simulink model "Marine_LocoMotive_UAV_est_git"  (R2018a)
settings: Solver=ode4  StartTime=0.0  StopTime=40  FixedStep=T  MaxStep=2*T  MinStep=T  RelTol=1e-4
values from neighbouring files (symbols this model uses):
  a_11 = 0.05*m_b    (= 0.625)    [Marine_LocoMotive_UAV_est_git_parameters.m]    (also in Marine_LocoMotive_UAV_medium_est_git_parameters.m = 1.6875; heave_dynamics_chart.m)
  a_33 = m_b    (= 12.5)    [Marine_LocoMotive_UAV_est_git_parameters.m]    (also in Marine_LocoMotive_UAV_medium_est_git_parameters.m = 33.75; heave_dynamics_chart.m)
  A_w = 1*3.3/2    (= 1.65)    [Marine_LocoMotive_UAV_est_git_parameters.m]    (also in Marine_LocoMotive_UAV_medium_est_git_parameters.m = 0.6)
  A_w2 = 1*1.2/2    (= 0.6)    [Marine_LocoMotive_UAV_est_git_parameters.m]    (also in Marine_LocoMotive_UAV_medium_est_git_parameters.m = 0.305)
  Ac = 0.0331    [Marine_LocoMotive_UAV_est_git_parameters.m]    (also in Marine_LocoMotive_UAV_medium_est_git_parameters.m = 0.422)
  alpha_bar = pi/4    (= 0.785398163397)    [Marine_LocoMotive_UAV_est_git_parameters.m]    (also in Marine_LocoMotive_UAV_medium_est_git_parameters.m; heave_dynamics_chart.m = pi/4*sign(V_bar(j)))
  Am = sysd.denominator{1}    [Marine_LocoMotive_UAV_est_git_parameters.m]    (also in Marine_LocoMotive_UAV_medium_est_git_parameters.m)
  Am1_LPF = sysd.denominator{1}    [Marine_LocoMotive_UAV_est_git_parameters.m]    (also in Marine_LocoMotive_UAV_medium_est_git_parameters.m)
  Am2_LPF = sysd.denominator{1}    [Marine_LocoMotive_UAV_est_git_parameters.m]    (also in Marine_LocoMotive_UAV_medium_est_git_parameters.m)
  Am_asw_LPF = sysd.denominator{1}    [Marine_LocoMotive_UAV_est_git_parameters.m]    (also in Marine_LocoMotive_UAV_medium_est_git_parameters.m)
  Am_coup_LPF = sysd.denominator{1}    [Marine_LocoMotive_UAV_est_git_parameters.m]    (also in Marine_LocoMotive_UAV_medium_est_git_parameters.m)
  Am_fast_coup_LPF = sysd.denominator{1}    [Marine_LocoMotive_UAV_est_git_parameters.m]    (also in Marine_LocoMotive_UAV_medium_est_git_parameters.m)
  Am_rdeL_LPF = sysd.denominator{1}    [Marine_LocoMotive_UAV_est_git_parameters.m]    (also in Marine_LocoMotive_UAV_medium_est_git_parameters.m)
  Am_reL_LPF = sysd.denominator{1}    [Marine_LocoMotive_UAV_est_git_parameters.m]    (also in Marine_LocoMotive_UAV_medium_est_git_parameters.m)
  Am_rref20_LPF = sysd.denominator{1}    [Marine_LocoMotive_UAV_est_git_parameters.m]    (also in Marine_LocoMotive_UAV_medium_est_git_parameters.m)
  Am_rref_LPF = sysd.denominator{1}    [Marine_LocoMotive_UAV_est_git_parameters.m]    (also in Marine_LocoMotive_UAV_medium_est_git_parameters.m)
  AmAlpha_LPF = sysd.denominator{1}    [Marine_LocoMotive_UAV_est_git_parameters.m]    (also in Marine_LocoMotive_UAV_medium_est_git_parameters.m)
  Amp_sf = 3    [Marine_LocoMotive_UAV_est_git_parameters.m]    (also in Marine_LocoMotive_UAV_medium_est_git_parameters.m)
  Amp_sf_rp = 0.05*m_u*g    (= 0.8829)    [Marine_LocoMotive_UAV_est_git_parameters.m]    (also in Marine_LocoMotive_UAV_medium_est_git_parameters.m = 9.56475)
  AmV_LPF = sysd.denominator{1}    [Marine_LocoMotive_UAV_est_git_parameters.m]    (also in Marine_LocoMotive_UAV_medium_est_git_parameters.m)
  AmZ_LPF = sysd.denominator{1}    [Marine_LocoMotive_UAV_est_git_parameters.m]    (also in Marine_LocoMotive_UAV_medium_est_git_parameters.m)
  b_11 = 0    [Marine_LocoMotive_UAV_est_git_parameters.m]    (also in Marine_LocoMotive_UAV_medium_est_git_parameters.m; heave_dynamics_chart.m)
  b_33 = 2*m_b*omega_h    (= 19.6349540849)    [Marine_LocoMotive_UAV_est_git_parameters.m]    (also in Marine_LocoMotive_UAV_medium_est_git_parameters.m = 84.8230016469; buoyancy_calc.m = 4.18879020479; heave_dynamics_chart.m = 2*m_b*omega_h)
  Bm = sysd.numerator{1}    [Marine_LocoMotive_UAV_est_git_parameters.m]    (also in Marine_LocoMotive_UAV_medium_est_git_parameters.m)
  Bm1_LPF = sysd.numerator{1}    [Marine_LocoMotive_UAV_est_git_parameters.m]    (also in Marine_LocoMotive_UAV_medium_est_git_parameters.m)
  Bm2_LPF = sysd.numerator{1}    [Marine_LocoMotive_UAV_est_git_parameters.m]    (also in Marine_LocoMotive_UAV_medium_est_git_parameters.m)
  Bm_asw_LPF = sysd.numerator{1}    [Marine_LocoMotive_UAV_est_git_parameters.m]    (also in Marine_LocoMotive_UAV_medium_est_git_parameters.m)
  Bm_coup_LPF = sysd.numerator{1}    [Marine_LocoMotive_UAV_est_git_parameters.m]    (also in Marine_LocoMotive_UAV_medium_est_git_parameters.m)
  Bm_fast_coup_LPF = sysd.numerator{1}    [Marine_LocoMotive_UAV_est_git_parameters.m]    (also in Marine_LocoMotive_UAV_medium_est_git_parameters.m)
  Bm_rdeL_LPF = sysd.numerator{1}    [Marine_LocoMotive_UAV_est_git_parameters.m]    (also in Marine_LocoMotive_UAV_medium_est_git_parameters.m)
  Bm_reL_LPF = sysd.numerator{1}    [Marine_LocoMotive_UAV_est_git_parameters.m]    (also in Marine_LocoMotive_UAV_medium_est_git_parameters.m)
  Bm_rref20_LPF = sysd.numerator{1}    [Marine_LocoMotive_UAV_est_git_parameters.m]    (also in Marine_LocoMotive_UAV_medium_est_git_parameters.m)
  Bm_rref_LPF = sysd.numerator{1}    [Marine_LocoMotive_UAV_est_git_parameters.m]    (also in Marine_LocoMotive_UAV_medium_est_git_parameters.m)
  BmAlpha_LPF = sysd.numerator{1}    [Marine_LocoMotive_UAV_est_git_parameters.m]    (also in Marine_LocoMotive_UAV_medium_est_git_parameters.m)
  BmV_LPF = sysd.numerator{1}    [Marine_LocoMotive_UAV_est_git_parameters.m]    (also in Marine_LocoMotive_UAV_medium_est_git_parameters.m)
  BmZ_LPF = sysd.numerator{1}    [Marine_LocoMotive_UAV_est_git_parameters.m]    (also in Marine_LocoMotive_UAV_medium_est_git_parameters.m)
  C_S = [5;9]*10^-3    [Marine_LocoMotive_UAV_est_git_parameters.m]    (also in Marine_LocoMotive_UAV_medium_est_git_parameters.m; heave_dynamics_chart.m = 0.075/(log10(Re)-2)^2)
  Cd_u = 0.2    [Marine_LocoMotive_UAV_est_git_parameters.m]    (also in Marine_LocoMotive_UAV_medium_est_git_parameters.m)
  D_x = b_11 + D_s(1)    [Marine_LocoMotive_UAV_est_git_parameters.m]    (also in Marine_LocoMotive_UAV_medium_est_git_parameters.m; heave_dynamics_chart.m = b_11 + D_s(i,j))
  D_z = b_33 + D_s(2)    [Marine_LocoMotive_UAV_est_git_parameters.m]    (also in Marine_LocoMotive_UAV_medium_est_git_parameters.m; heave_dynamics_chart.m)
  dc_M_p = 6.7    [Marine_LocoMotive_UAV_est_git_parameters.m]    (also in Marine_LocoMotive_UAV_medium_est_git_parameters.m)
  Delta_h = (A_im/A_b-0.5)*h_b    (= -0.0625)    [Marine_LocoMotive_UAV_est_git_parameters.m]    (also in Marine_LocoMotive_UAV_medium_est_git_parameters.m = -0.075; heave_dynamics_chart.m)
  eps_V = 0.1    [Marine_LocoMotive_UAV_est_git_parameters.m]    (also in Marine_LocoMotive_UAV_medium_est_git_parameters.m)
  epsilon_1 = 5    [Marine_LocoMotive_UAV_est_git_parameters.m]    (also in Marine_LocoMotive_UAV_medium_est_git_parameters.m)
  epsilon_e_u1 = 0.05    [Marine_LocoMotive_UAV_est_git_parameters.m]    (also in Marine_LocoMotive_UAV_medium_est_git_parameters.m)
  epsilon_w = 0    [Marine_LocoMotive_UAV_est_git_parameters.m]    (also in Marine_LocoMotive_UAV_medium_est_git_parameters.m)
  epsilon_w2 = pi    (= 3.14159265359)    [Marine_LocoMotive_UAV_est_git_parameters.m]    (also in Marine_LocoMotive_UAV_medium_est_git_parameters.m)
  g = 9.81    [Marine_LocoMotive_UAV_est_git_parameters.m]    (also in Marine_LocoMotive_UAV_medium_est_git_parameters.m; heave_dynamics_chart.m)
  gamma_d_p = (2*0.3/0.03*2*0.2*12/4)/10    (= 2.4)    [Marine_LocoMotive_UAV_est_git_parameters.m]    (also in Marine_LocoMotive_UAV_medium_est_git_parameters.m)
  H = 10    [Marine_LocoMotive_UAV_est_git_parameters.m]    (also in Marine_LocoMotive_UAV_medium_est_git_parameters.m)
  h_b = 0.25    [Marine_LocoMotive_UAV_est_git_parameters.m]    (also in Marine_LocoMotive_UAV_medium_est_git_parameters.m = 0.3; buoyancy_calc.m = 0.15; heave_dynamics_chart.m)
  J_b = m_b*h_b*l_b/12    (= 0.208333333333)    [Marine_LocoMotive_UAV_est_git_parameters.m]    (also in Marine_LocoMotive_UAV_medium_est_git_parameters.m = 1.265625; heave_dynamics_chart.m)
  J_u = 0.03    [Marine_LocoMotive_UAV_est_git_parameters.m]    (also in Marine_LocoMotive_UAV_medium_est_git_parameters.m = 1.51708333333)
  K = 40    [Marine_LocoMotive_UAV_est_git_parameters.m]    (also in Marine_LocoMotive_UAV_medium_est_git_parameters.m = 83.3333333333)
  k3 = 24    [Marine_LocoMotive_UAV_est_git_parameters.m]    (also in Marine_LocoMotive_UAV_medium_est_git_parameters.m)
  k4 = 0.8    [Marine_LocoMotive_UAV_est_git_parameters.m]    (also in Marine_LocoMotive_UAV_medium_est_git_parameters.m)
  k_w = omega_w^2/g    (= 0.0628797426165)    [Marine_LocoMotive_UAV_est_git_parameters.m]    (also in Marine_LocoMotive_UAV_medium_est_git_parameters.m = 0.160972141098; heave_dynamics_chart.m = omega_w^2/g)
  k_w2 = omega_w2^2/g    (= 0.160972141098)    [Marine_LocoMotive_UAV_est_git_parameters.m]    (also in Marine_LocoMotive_UAV_medium_est_git_parameters.m = 0.251518970466)
  kd_a = 5.6    [Marine_LocoMotive_UAV_est_git_parameters.m]    (also in Marine_LocoMotive_UAV_medium_est_git_parameters.m)
  kd_r = 19.5    [Marine_LocoMotive_UAV_est_git_parameters.m]    (also in Marine_LocoMotive_UAV_medium_est_git_parameters.m)
  kd_t = 10    [Marine_LocoMotive_UAV_est_git_parameters.m]    (also in Marine_LocoMotive_UAV_medium_est_git_parameters.m = 25)
  kd_x = 5    [Marine_LocoMotive_UAV_est_git_parameters.m]    (also in Marine_LocoMotive_UAV_medium_est_git_parameters.m)
  kd_z = 2    [Marine_LocoMotive_UAV_est_git_parameters.m]    (also in Marine_LocoMotive_UAV_medium_est_git_parameters.m)
  ki_a = 1.6    [Marine_LocoMotive_UAV_est_git_parameters.m]    (also in Marine_LocoMotive_UAV_medium_est_git_parameters.m)
  ki_r = 9    [Marine_LocoMotive_UAV_est_git_parameters.m]    (also in Marine_LocoMotive_UAV_medium_est_git_parameters.m)
  ki_T = 12    [Marine_LocoMotive_UAV_est_git_parameters.m]    (also in Marine_LocoMotive_UAV_medium_est_git_parameters.m)
  ki_x = 1.2    [Marine_LocoMotive_UAV_est_git_parameters.m]    (also in Marine_LocoMotive_UAV_medium_est_git_parameters.m)
  ki_z = 1    [Marine_LocoMotive_UAV_est_git_parameters.m]    (also in Marine_LocoMotive_UAV_medium_est_git_parameters.m)
  kp_a = 9.6    [Marine_LocoMotive_UAV_est_git_parameters.m]    (also in Marine_LocoMotive_UAV_medium_est_git_parameters.m)
  kp_r = 45    [Marine_LocoMotive_UAV_est_git_parameters.m]    (also in Marine_LocoMotive_UAV_medium_est_git_parameters.m)
  kp_t = 20    [Marine_LocoMotive_UAV_est_git_parameters.m]    (also in Marine_LocoMotive_UAV_medium_est_git_parameters.m = 50)
  kp_T = 25    [Marine_LocoMotive_UAV_est_git_parameters.m]    (also in Marine_LocoMotive_UAV_medium_est_git_parameters.m)
  kp_x = 7    [Marine_LocoMotive_UAV_est_git_parameters.m]    (also in Marine_LocoMotive_UAV_medium_est_git_parameters.m)
  kp_z = 3    [Marine_LocoMotive_UAV_est_git_parameters.m]    (also in Marine_LocoMotive_UAV_medium_est_git_parameters.m)
  L = 0.2    [Marine_LocoMotive_UAV_est_git_parameters.m]    (also in Marine_LocoMotive_UAV_medium_est_git_parameters.m = 0.8)
  l_b = 0.8    [Marine_LocoMotive_UAV_est_git_parameters.m]    (also in Marine_LocoMotive_UAV_medium_est_git_parameters.m = 1.5; buoyancy_calc.m = 0.5; heave_dynamics_chart.m)
  Lc_0 = 7    [Marine_LocoMotive_UAV_est_git_parameters.m]    (also in Marine_LocoMotive_UAV_medium_est_git_parameters.m = 20)
  LIMIT_CMD_PITCH = 45*pi/180    (= 0.785398163397)    [Marine_LocoMotive_UAV_est_git_parameters.m]    (also in Marine_LocoMotive_UAV_medium_est_git_parameters.m)
  LIMIT_uCMD_HEIGHT = 0.9*n_motors*K    (= 144)    [Marine_LocoMotive_UAV_est_git_parameters.m]    (also in Marine_LocoMotive_UAV_medium_est_git_parameters.m = 450)
  m_b = rho_w*Vol_b/4    (= 12.5)    [Marine_LocoMotive_UAV_est_git_parameters.m]    (also in Marine_LocoMotive_UAV_medium_est_git_parameters.m = 33.75; buoyancy_calc.m = 5; heave_dynamics_chart.m)
  m_u = 1.8    [Marine_LocoMotive_UAV_est_git_parameters.m]    (also in Marine_LocoMotive_UAV_medium_est_git_parameters.m = 19.5)
  min_sf = 5    [Marine_LocoMotive_UAV_est_git_parameters.m]    (also in Marine_LocoMotive_UAV_medium_est_git_parameters.m)
  min_sf_rp = 0.35*m_u*g    (= 6.1803)    [Marine_LocoMotive_UAV_est_git_parameters.m]    (also in Marine_LocoMotive_UAV_medium_est_git_parameters.m = 66.95325)
  n_motors = 4    [Marine_LocoMotive_UAV_est_git_parameters.m]    (also in Marine_LocoMotive_UAV_medium_est_git_parameters.m = 6)
  nu_w = 1.787*10^-6    (= 1.787e-06)    [Marine_LocoMotive_UAV_est_git_parameters.m]    (also in Marine_LocoMotive_UAV_medium_est_git_parameters.m; buoyancy_calc.m; heave_dynamics_chart.m)
  omega_w = 2*pi/T_w    (= 0.785398163397)    [Marine_LocoMotive_UAV_est_git_parameters.m]    (also in Marine_LocoMotive_UAV_medium_est_git_parameters.m = 1.25663706144; heave_dynamics_chart.m = 2*pi/T_i)
  omega_w2 = 2*pi/T_w2    (= 1.25663706144)    [Marine_LocoMotive_UAV_est_git_parameters.m]    (also in Marine_LocoMotive_UAV_medium_est_git_parameters.m = 1.57079632679)
  r_0 = sqrt( (X0_b(1) - X0_u(1))^2 +(X0_b(2) - X0_u(2))^2 )    [Marine_LocoMotive_UAV_est_git_parameters.m]    (also in Marine_LocoMotive_UAV_medium_est_git_parameters.m)
  R_b = 0.1    [buoyancy_calc.m]
  r_bar = Lc_0-0.3    (= 6.7)    [Marine_LocoMotive_UAV_est_git_parameters.m]    (also in Marine_LocoMotive_UAV_medium_est_git_parameters.m = 19.7)
  r_min = (zu_bar-H)-0.2    [Marine_LocoMotive_UAV_est_git_parameters.m]    (also in Marine_LocoMotive_UAV_medium_est_git_parameters.m)
  rho_a = 1.225    [Marine_LocoMotive_UAV_est_git_parameters.m]    (also in Marine_LocoMotive_UAV_medium_est_git_parameters.m)
  rho_w = 1000    [Marine_LocoMotive_UAV_est_git_parameters.m]    (also in Marine_LocoMotive_UAV_medium_est_git_parameters.m; buoyancy_calc.m; heave_dynamics_chart.m)
  T = 1/500    (= 0.002)    [Marine_LocoMotive_UAV_est_git_parameters.m]    (also in Marine_LocoMotive_UAV_medium_est_git_parameters.m)
  T_init = 10    [Marine_LocoMotive_UAV_est_git_parameters.m]    (also in Marine_LocoMotive_UAV_medium_est_git_parameters.m)
  Theta0 = 0    [Marine_LocoMotive_UAV_est_git_parameters.m]    (also in Marine_LocoMotive_UAV_medium_est_git_parameters.m)
  torque_corr = 2*cosd(60)+1    [Marine_LocoMotive_UAV_est_git_parameters.m]    (also in Marine_LocoMotive_UAV_medium_est_git_parameters.m)
  u_s = w_dir*A_w^2*omega_w*k_w*exp(2*k_w*(-Delta_h/2))    [Marine_LocoMotive_UAV_est_git_parameters.m]    (also in Marine_LocoMotive_UAV_medium_est_git_parameters.m)
  u_s2 = w_dir2*A_w2^2*omega_w2*k_w2*exp(2*k_w2*(-Delta_h/2))    [Marine_LocoMotive_UAV_est_git_parameters.m]    (also in Marine_LocoMotive_UAV_medium_est_git_parameters.m)
  u_t = -1*0.5*1    (= -0.5)    [Marine_LocoMotive_UAV_est_git_parameters.m]    (also in Marine_LocoMotive_UAV_medium_est_git_parameters.m)
  u_w = 0*0.2    (= 0)    [Marine_LocoMotive_UAV_est_git_parameters.m]    (also in Marine_LocoMotive_UAV_medium_est_git_parameters.m)
  V0_b = [u_t+u_w+u_s+v_x_w, v_z_w].*[1 1]    [Marine_LocoMotive_UAV_est_git_parameters.m]    (also in Marine_LocoMotive_UAV_medium_est_git_parameters.m = [u_t+u_w+u_s+v_x_w, v_z_w])
  V0_u = V0_b    [Marine_LocoMotive_UAV_est_git_parameters.m]    (also in Marine_LocoMotive_UAV_medium_est_git_parameters.m = [0 0])
  V_bar = 4    [Marine_LocoMotive_UAV_est_git_parameters.m]    (also in Marine_LocoMotive_UAV_medium_est_git_parameters.m; heave_dynamics_chart.m = [-20:0.1:20]')
  Vol_b = A_b*l_b    (= 0.05)    [Marine_LocoMotive_UAV_est_git_parameters.m]    (also in Marine_LocoMotive_UAV_medium_est_git_parameters.m = 0.135; heave_dynamics_chart.m)
  w_dir = 1    [Marine_LocoMotive_UAV_est_git_parameters.m]    (also in Marine_LocoMotive_UAV_medium_est_git_parameters.m; heave_dynamics_chart.m)
  w_dir2 = 1    [Marine_LocoMotive_UAV_est_git_parameters.m]    (also in Marine_LocoMotive_UAV_medium_est_git_parameters.m)
  X0_b = [0,H-Delta_h]    [Marine_LocoMotive_UAV_est_git_parameters.m]    (also in Marine_LocoMotive_UAV_medium_est_git_parameters.m)
  X0_u = X0_b + [3/7 3/7]*Lc_0    [Marine_LocoMotive_UAV_est_git_parameters.m]    (also in Marine_LocoMotive_UAV_medium_est_git_parameters.m)
  zu_bar = X0_b(2) + Lc_0*sin(alpha_bar_0)    [Marine_LocoMotive_UAV_est_git_parameters.m]    (also in Marine_LocoMotive_UAV_medium_est_git_parameters.m)
undefined symbols (not defined in the file or in its folder): Am_HPF, Am_LPF, Am_LPF2, an1, an1_v, an2, an3, Bm_HPF, Bm_LPF, Bm_LPF2, bn1, bn1_v, bn2, bn3, DiscIntNeverNeededParam, F, Light, magnitude, MIL, OMEGA_FILTER_OUTER, Tc, Tg, Tn, Ts, Tsc, Tz, X_GPS_offset
libraries: simulink x55, simulink_extras x9, aerolibwind2 x2
(part 2 of 9)

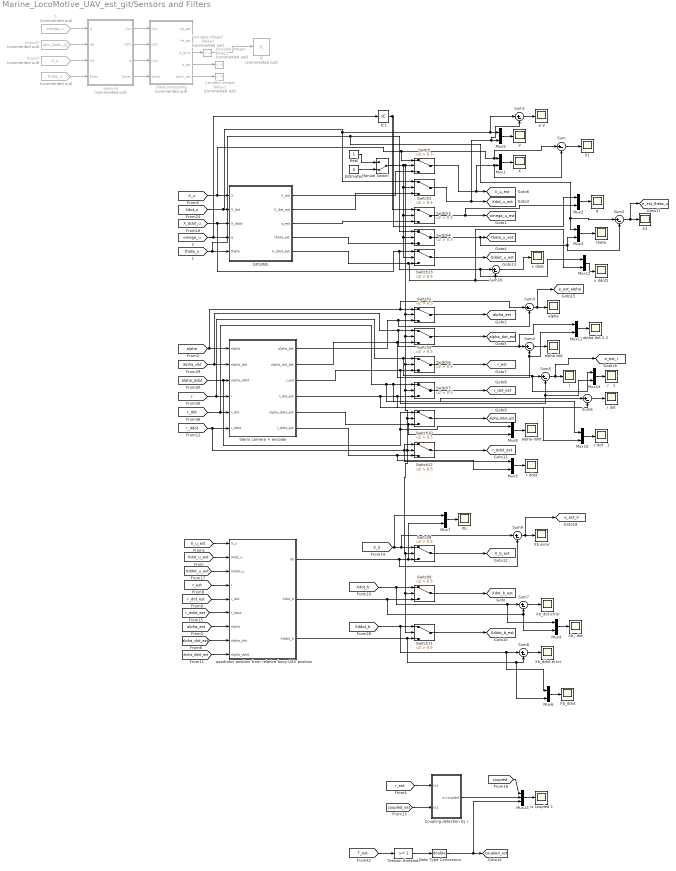
== system Marine_LocoMotive_UAV_est_git/Sensors and Filters ==
  "    " : From  Commented=on  GotoTag=theta_u  TagVisibility=global
  "   1" : From  Commented=on  GotoTag=omega_u  TagVisibility=global
  Coupling detection by r : Subsystem
  Data Type Conversion : DataTypeConversion  OutDataTypeStr=double
  Data processing : Subsystem  Commented=on
  Estimates : Constant  Value=0
  From37 : From  Commented=on  GotoTag=acc_body_u  TagVisibility=global
  From7 : From  Commented=on  GotoTag=X_u  TagVisibility=global
  GPS/INS : Subsystem
  IC : InitialCondition  Commented=on  Value=0
  IC1 : InitialCondition  Value=0
  Manual Switch : ManualSwitch  CurrentSetting=0
  Mux{1..12,14} (13 alike) : Mux  Inputs=2
  Mux13 : Mux  Inputs=3
  Real : Constant
  Sensors : Subsystem  Commented=on
  Sterio camera + encoder : Subsystem
  Sum{,1..10} (11 alike) : Sum  Inputs=|+-
  Switch{,1..13} (14 alike) : Switch  Criteria=u2 > Threshold  Threshold=0.5
  Tension threshold : simulink/Logic and Bit Operations/Compare To Constant  relop=>=  const=1  OutDataTypeStr=boolean
  V : Scope
  Variable Integer Delay1 : Delay  Commented=on  DelayLength=0
  Variable Integer Delay2 : Delay  Commented=on  DelayLength=0
  Variable Integer Delay3 : Delay  Commented=on  DelayLength=0
  X : Scope
  X1 : Scope
  X3 : Scope
  "Xb " : Scope
  Xb error : Scope
  "Xb_ dot " : Scope
  "Xb_ddot " : Scope
  "Xb_ddot error  " : Scope
  Xb_dot error : Scope
  "alpha  " : Scope
  "alpha ddot " : Scope
  "alpha dot " : Scope
  alpha dot 2 2 : Scope
  e V : Scope
  is coupled 1 : Scope
  q : Scope
  quadrotor position from relative buoy-UAV position : Subsystem
  "r   " : Scope
  r   1 : Scope
  "r ddot   " : Scope
  "r dot  " : Scope
  r dot   1 : Scope
  theta : Scope
  x ddot : Scope
  x ddot1 : Scope
  tag scope: X_b_est=global, X_u_est=global, Xddot_b_est=global, Xddot_u_est=global, Xdot_b_est=global, Xdot_u_est=global, alpha_ddot_est=global, alpha_dot_est=global, alpha_est=global, coupled_est=global, e_est_V=global, e_est_alpha=global, e_est_r=global, e_est_theta_u=global, omega_u_est=global, r_ddot_est=global, r_dot_est=global, r_est=global, theta_u_est=global
  wires:
  Data processing/4("q_est ") -> Variable Integer Delay1/1
  "    "/1 -> Sensors/4(Euler)
  Sensors/3(" q") -> Data processing/3(p,q,r)
  "   1"/1 -> Sensors/1("q ")
  From7/1 -> Sensors/3(Xe)
  Sensors/1(Acc) -> Data processing/1(Acc)
  Sensors/2(GPS) -> Data processing/2("GPS ")
  From37/1 -> Sensors/2(Ab)
  Data processing/3(q_gyro) -> Variable Integer Delay3/1
  Data processing/5(pitch_est) -> Variable Integer Delay2/1
  Sensors/4(Sonar) -> Data processing/4(Sonar)
  Estimates/1 -> Manual Switch/2
  Real/1 -> Manual Switch/1
  Switch/1 -> Sum/2, Mux1/2, [X_u_est]
  Switch1/1 -> Sum1/2, Mux5/2, [Xdot_u_est]
  Switch3/1 -> Mux2/2, [omega_u_est]
  Switch4/1 -> Mux3/2, Sum2/2, [theta_u_est]
  GPS/INS/1(X_est) -> Switch/3
  GPS/INS/2(X_dot_est) -> Switch1/3
  Variable Integer Delay3/1 -> IC/1
  [X_u] -> Sum/1, Mux1/1, Switch/1, GPS/INS/1(X)
  [omega_u] -> IC1/1, GPS/INS/4(q)
  [Xdot_u] -> Sum1/1, Mux5/1, Switch1/1, GPS/INS/2(X_dot)
  GPS/INS/4(theta_est) -> Switch4/3
  GPS/INS/3(q_est) -> Switch3/3
  IC1/1 -> Mux2/1, Switch3/1
  [theta_u] -> Sum2/1, Mux3/1, Switch4/1, GPS/INS/5(theta)
  Mux5/1 -> V/1
  Mux1/1 -> X/1
  Mux2/1 -> q/1
  Mux3/1 -> theta/1
  Sum/1 -> X1/1
  Sum1/1 -> e V/1
  Sum2/1 -> [e_est_theta_u], X3/1
  [alpha_dot] -> Mux11/1, Sum4/1, Switch5/1, Sterio camera + encoder/2(alpha_dot)
  [r] -> Mux14/1, Sum5/1, Switch6/1, Sterio camera + encoder/4(r)
  [r_dot] -> Mux10/1, Sum6/1, Switch7/1, Sterio camera + encoder/5(r_dot)
  Sterio camera + encoder/2(alpha_dot_est) -> Mux11/2, Sum4/2, Switch5/3
  Sterio camera + encoder/3(r_est) -> Sum5/2, Mux14/2, Switch6/3
  Switch2/1 -> [alpha_est]
  Switch5/1 -> [alpha_dot_est]
  Switch6/1 -> [r_est]
  Switch7/1 -> [r_dot_est]
  Sum3/1 -> [e_est_alpha], "alpha  "/1
  [alpha] -> Sum3/1, Switch2/1, Sterio camera + encoder/1(alpha)
  Sterio camera + encoder/1(alpha_est) -> Sum3/2, Switch2/3
  Sum4/1 -> "alpha dot "/1
  Sum5/1 -> [e_est_r], "r   "/1
  Sterio camera + encoder/4(r_dot_est) -> Mux10/2, Sum6/2, Switch7/3
  Sum6/1 -> "r dot  "/1
  [X_u_est] -> quadrotor position from relative buoy-UAV position/1(X_u)
  [Xdot_u_est] -> quadrotor position from relative buoy-UAV position/2(Xdot_u)
  [r_est] -> quadrotor position from relative buoy-UAV position/4(r)
  [r_dot_est] -> quadrotor position from relative buoy-UAV position/5(r_dot)
  [alpha_est] -> quadrotor position from relative buoy-UAV position/7(alpha)
  [alpha_dot_est] -> quadrotor position from relative buoy-UAV position/8(alpha_dot)
  quadrotor position from relative buoy-UAV position/2(Xdot_b) -> Mux4/2, Sum7/2, Switch9/3
  quadrotor position from relative buoy-UAV position/1(Xb) -> Sum9/2, Mux7/2, Switch8/3
  [alpha_ddot] -> Switch10/1, Mux8/1, Sterio camera + encoder/3(alpha_ddot)
  Sterio camera + encoder/5(alpha_ddot_est) -> Mux8/2, Switch10/3
  Switch10/1 -> [alpha_ddot_est]
  [Xdot_b] -> Mux4/1, Sum7/1, Switch9/1
  [alpha_ddot_est] -> quadrotor position from relative buoy-UAV position/9(alpha_ddot)
  [Xddot_u_est] -> quadrotor position from relative buoy-UAV position/3(Xddot_u)
  quadrotor position from relative buoy-UAV position/3(Xddot_b) -> Mux6/2, Sum8/2, Switch11/3
  [r_ddot] -> Mux9/1, Switch12/1, Sterio camera + encoder/6(r_ddot)
  Switch12/1 -> [r_ddot_est]
  Switch9/1 -> [Xdot_b_est]
  Switch11/1 -> [Xddot_b_est]
  Sum7/1 -> Xb_dot error/1
  Manual Switch/1 -> Switch10/2, Switch12/2, Switch8/2, Switch11/2, Switch9/2, Switch7/2, Switch6/2, Switch5/2, Switch2/2, Switch/2, Switch13/2, Switch4/2, Switch3/2, Switch1/2
  Sum8/1 -> "Xb_ddot error  "/1
  Sum9/1 -> [e_est_V], Xb error/1
  Switch8/1 -> [X_b_est]
  [X_b] -> Mux7/1, Sum9/1, Switch8/1
  Mux4/1 -> "Xb_ dot "/1
  Mux6/1 -> "Xb_ddot "/1
  [Xddot_b] -> Mux6/1, Sum8/1, Switch11/1
  [r_ddot_est] -> quadrotor position from relative buoy-UAV position/6(r_ddot)
  [X_ddot_u] -> Mux12/1, Sum10/1, Switch13/1, GPS/INS/3(X_ddot)
  Switch13/1 -> [Xddot_u_est]
  Mux7/1 -> "Xb "/1
  Mux8/1 -> "alpha ddot "/1
  Mux9/1 -> "r ddot   "/1
  Sterio camera + encoder/6(r_ddot_est) -> Mux9/2, Switch12/3
  Sum10/1 -> x ddot/1
  Mux10/1 -> r dot   1/1
  Mux11/1 -> alpha dot 2 2/1
  GPS/INS/5(X_ddot_est) -> Mux12/2, Sum10/2, Switch13/3
  Mux12/1 -> x ddot1/1
  Mux13/1 -> is coupled 1/1
  Mux14/1 -> r   1/1
  [r_est] -> Coupling detection by r/1(In1)
  [coupled_est] -> Coupling detection by r/2(In2)
  [T_est] -> Tension threshold/1
  Tension threshold/1 -> Data Type Conversion/1
  Data Type Conversion/1 -> Mux13/3, [coupled_est]
  Coupling detection by r/1(is coupled) -> Mux13/2
  [coupled] -> Mux13/1

== system Marine_LocoMotive_UAV_est_git/Subsystem ==

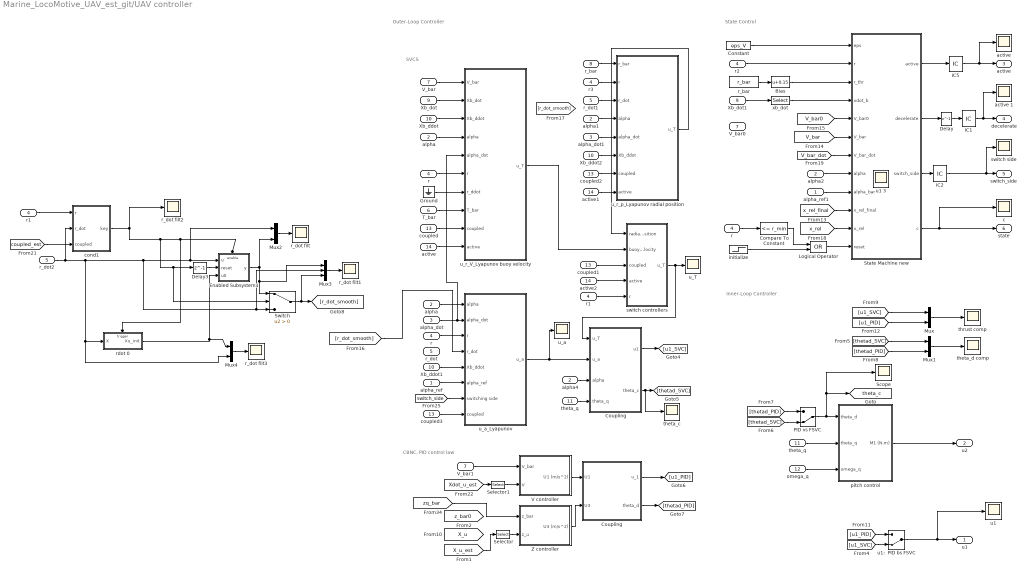
== system Marine_LocoMotive_UAV_est_git/UAV controller ==
  note: State Control
  note: Inner-Loop Controller
  note: Outer-Loop Controller
  note: CBNC, PID control law
  note: SVCS
  alpha_ref : Inport
  alpha : Inport  Port=2
  alpha_dot : Inport  Port=3
  r : Inport  Port=4
  r_dot : Inport  Port=5
  T_bar : Inport  Port=6
  V_bar : Inport  Port=7
  r_bar : Inport  Port=8
  Xb_dot : Inport  Port=9
  Xb_ddot : Inport  Port=10
  theta_q : Inport  Port=11
  omega_q : Inport  Port=12
  coupled : Inport  Port=13
  active : Inport  Port=14
  " active " : Scope
  " active 1" : Scope
  " c " : Scope
  " r" : InportShadow  Port=4
  " r1" : InportShadow  Port=4
  Bias : Bias  Bias=0.15
  Compare To Constant : simulink/Logic and Bit Operations/Compare To Constant  relop=<=  const=r_min  OutDataTypeStr=boolean
  Constant : Constant  Value=eps_V
  Coupling : Subsystem
  "Coupling " : Subsystem
  Delay : Delay  DelayLength=1  InitialCondition=0
  Delay3 : Delay  DelayLength=1  InitialCondition=0
  Enabled Subsystem1 : Subsystem  TreatAsAtomicUnit=on
  Ground : Ground
  IC1 : InitialCondition  Value=0
  IC2 : InitialCondition  Value=0
  IC5 : InitialCondition  Value=0
  Logical Operator : Logic  Operator=OR  AllPortsSameDT=off  OutDataTypeStr=boolean
  Mux{,1..2,4} (4 alike) : Mux  Inputs=2
  Mux3 : Mux  Inputs=3
  PID vs FSVC : ManualSwitch  CurrentSetting=0
  Scope : Scope
  Selector : Selector  InputPortWidth=2  IndexOptions=Index vector (dialog)  Indices=2  OutputSizes=1
  Selector1 : Selector  InputPortWidth=2  IndexOptions=Index vector (dialog)  Indices=1  OutputSizes=1
  State Machine new : MATLAB Function  TreatAsAtomicUnit=on
  Switch : Switch  Criteria=u2 > Threshold
  V controller : Subsystem
  V_bar0 : InportShadow  Port=7
  V_bar1 : InportShadow  Port=7
  Xb_ddot1 : InportShadow  Port=10
  Xb_ddot2 : InportShadow  Port=10
  Xb_dot1 : InportShadow  Port=9
  Z controller : Subsystem
  active1 : InportShadow  Port=14
  active2 : InportShadow  Port=14
  "alpha " : InportShadow  Port=2
  alpha1 : InportShadow  Port=2
  alpha2 : InportShadow  Port=2
  alpha4 : InportShadow  Port=2
  alpha_dot1 : InportShadow  Port=3
  alpha_ref1 : InportShadow
  cond1 : Subsystem
  coupled1 : InportShadow  Port=13
  coupled2 : InportShadow  Port=13
  coupled3 : InportShadow  Port=13
  initialize : Step  Time=T_init  Before=1  After=0  SampleTime=0
  pitch control : Subsystem
  "r " : InportShadow  Port=4
  r1 : InportShadow  Port=4
  r2 : InportShadow  Port=4
  r3 : InportShadow  Port=4
  "r_bar " : Constant  Value=r_bar
  r_dot filt{,1..3} (4 alike) : Scope
  r_dot1 : InportShadow  Port=5
  r_dot2 : InportShadow  Port=5
  rdot 0 : Subsystem  TreatAsAtomicUnit=on
  switch controllers : Subsystem
  "switch side  " : Scope
  "theta_c " : Scope
  theta_d comp : Scope
  "theta_q " : InportShadow  Port=11
  thrust comp : Scope
  "u1 " : Scope
  u1 3 : Scope
  u1:  PID bs FSVC : ManualSwitch  CurrentSetting=0
  u_T : Scope
  u_a : Scope
  u_a_Lyapunov : Subsystem
  u_r_V_Lyapunov buoy velocity : Subsystem
  u_r_p_Lyapunov radial position : Subsystem
  xb_dot : Selector  InputPortWidth=2  IndexOptions=Index vector (dialog)  Indices=1  OutputSizes=1
  u1 : Outport
  u2 : Outport  Port=2
  " active" : Outport  Port=3
  " decelerate" : Outport  Port=4
  " switch_side" : Outport  Port=5
  state : Outport  Port=6
  tag scope: theta_c=global
  wires:
  theta_q/1 -> pitch control/2(theta_q)
  omega_q/1 -> pitch control/3(omega_q)
  pitch control/1(M1 (N.m)) -> u2/1
  alpha4/1 -> "Coupling "/3(alpha)
  PID vs FSVC/1 -> Scope/1, [theta_c], pitch control/1(theta_d)
  u1:  PID bs FSVC/1 -> "u1 "/1, u1/1
  alpha/1 -> u_r_V_Lyapunov buoy velocity/4(alpha)
  T_bar/1 -> u_r_V_Lyapunov buoy velocity/8(T_bar)
  V_bar/1 -> u_r_V_Lyapunov buoy velocity/1(V_bar)
  Xb_dot/1 -> u_r_V_Lyapunov buoy velocity/2(Xb_dot)
  Xb_ddot/1 -> u_r_V_Lyapunov buoy velocity/3(Xb_ddot)
  "alpha "/1 -> u_a_Lyapunov/1(alpha)
  Xb_ddot1/1 -> u_a_Lyapunov/5(Xb_ddot)
  alpha_ref/1 -> u_a_Lyapunov/6(alpha_ref)
  alpha_dot/1 -> u_r_V_Lyapunov buoy velocity/5(alpha_dot), u_a_Lyapunov/2("alpha_dot ")
  [zq_bar] -> Z controller/1(z_bar)
  Selector/1 -> Z controller/2(z_u)
  [X_u_est] -> Selector/1
  V_bar1/1 -> V controller/1(V_bar)
  [Xdot_u_est] -> Selector1/1
  Selector1/1 -> V controller/2(V)
  V controller/1(U1 (m/s^2)) -> Coupling/1(U1)
  Z controller/1(U3 (m/s^2)) -> Coupling/2(U3)
  Mux/1 -> thrust comp/1
  Mux1/1 -> theta_d comp/1
  [thetad_SVC] -> Mux1/1
  [u1_SVC] -> u1:  PID bs FSVC/2
  u_a_Lyapunov/1(u_a) -> u_a/1, "Coupling "/2(u_a)
  Xb_dot1/1 -> xb_dot/1
  [V_bar0] -> State Machine new/5(V_bar0)
  xb_dot/1 -> State Machine new/4(xdot_b)
  Constant/1 -> State Machine new/1(eps)
  State Machine new/1(active) -> IC5/1
  State Machine new/4(c) -> state/1, " c "/1
  IC5/1 -> " active "/1, " active"/1
  Coupling/1(u_1) -> [u1_PID]
  Coupling/2(theta_d) -> [thetad_PID]
  "Coupling "/1(u1) -> [u1_SVC]
  [thetad_SVC] -> PID vs FSVC/2
  [thetad_PID] -> PID vs FSVC/1
  [thetad_PID] -> Mux1/2
  [u1_SVC] -> Mux/1
  [u1_PID] -> u1:  PID bs FSVC/1
  [u1_PID] -> Mux/2
  "Coupling "/2(theta_c) -> [thetad_SVC], "theta_c "/1
  r_bar/1 -> u_r_p_Lyapunov radial position/1("r_bar ")
  r/1 -> Compare To Constant/1
  Compare To Constant/1 -> Logical Operator/1
  initialize/1 -> Logical Operator/2
  active/1 -> u_r_V_Lyapunov buoy velocity/10(active)
  coupled/1 -> u_r_V_Lyapunov buoy velocity/9(coupled)
  Ground/1 -> u_r_V_Lyapunov buoy velocity/7(r_ddot)
  [r_dot_smooth] -> u_a_Lyapunov/4(r_dot)
  "r "/1 -> u_r_V_Lyapunov buoy velocity/6(r)
  " r"/1 -> u_a_Lyapunov/3(r)
  r3/1 -> u_r_p_Lyapunov radial position/2(r)
  r_dot1/1 -> u_r_p_Lyapunov radial position/3(r_dot)
  alpha1/1 -> u_r_p_Lyapunov radial position/4(alpha)
  alpha_dot1/1 -> u_r_p_Lyapunov radial position/5(alpha_dot)
  Xb_ddot2/1 -> u_r_p_Lyapunov radial position/6(Xb_ddot)
  active1/1 -> u_r_p_Lyapunov radial position/8(active)
  "r_bar "/1 -> Bias/1
  coupled2/1 -> u_r_p_Lyapunov radial position/7(coupled)
  switch controllers/1(u_T) -> "Coupling "/1(u_T), u_T/1
  u_r_V_Lyapunov buoy velocity/1(u_T) -> switch controllers/2(buoy velocity)
  coupled1/1 -> switch controllers/3(coupled)
  active2/1 -> switch controllers/4(active)
  u_r_p_Lyapunov radial position/1(u_T) -> switch controllers/1(radial position)
  State Machine new/2(decelerate) -> Delay/1
  IC1/1 -> " active 1"/1, " decelerate"/1
  alpha_ref1/1 -> State Machine new/9(alpha_bar)
  alpha2/1 -> State Machine new/8(alpha)
  State Machine new/3(switch_side) -> IC2/1
  IC2/1 -> "switch side  "/1, " switch_side"/1
  Logical Operator/1 -> State Machine new/12(reset)
  r1/1 -> switch controllers/5(r)
  [x_rel_final] -> State Machine new/10(x_rel_final)
  [switch_side] -> u_a_Lyapunov/7(switching side)
  Mux2/1 -> r_dot filt/1
  Enabled Subsystem1/1(y) -> Mux2/2, Mux3/1, Switch/1
  Switch/1 -> Mux3/3, [r_dot_smooth]
  Mux3/1 -> r_dot filt1/1
  [coupled_est] -> cond1/3(coupled)
  coupled3/1 -> u_a_Lyapunov/8(coupled)
  r_dot2/1 -> cond1/2(r_dot), Enabled Subsystem1/1(u), Mux2/1, Mux3/2, Switch/3, rdot 0/1(X), Mux4/2
  Mux4/1 -> r_dot filt3/1
  rdot 0/1(Xu_init) -> Mux4/1, Enabled Subsystem1/3(u0)
  " r1"/1 -> cond1/1(r)
  cond1/1(key) -> Delay3/1, Switch/2, rdot 0/Trigger, Enabled Subsystem1/Enable, r_dot filt2/1
  Delay3/1 -> Enabled Subsystem1/2(reset)
  [x_rel] -> State Machine new/11(x_rel)
  [V_bar] -> State Machine new/6(V_bar)
  Bias/1 -> State Machine new/3(r_thr)
  [V_bar_dot] -> State Machine new/7(V_bar_dot)
  Delay/1 -> IC1/1
  r2/1 -> State Machine new/2(r)
  "theta_q "/1 -> "Coupling "/4(theta_q)

== system Marine_LocoMotive_UAV_est_git/Wind model ==
  Bias : Bias  Bias=0.05
  Discrete Wind Gust Model : aerolibwind2/Discrete Wind Gust Model  units=Metric (MKS)  Gx=on  Gy=off  Gz=off  t_0=1  d_m=[1 1 80]  v_m=V_w
      settings: SourceProductName=Aerospace Blockset
  Dryden Wind Turbulence Model (Continuous (+q +r)) : aerolibwind2/Dryden Wind Turbulence Model  (Continuous (+q -r))  Commented=on  units=Metric (MKS)  spec=MIL-F-8785C  model=Continuous Dryden (+q +r)  W20=20  Wdeg=30  TurbProb=10^-2 - Light  L_high=533.4  Wingspan=1.5  ts=0.02  Seed=[11341 23342 13423 13344]  T_on=on
      settings: SourceProductName=Aerospace Blockset
  From25 : From  Commented=on  GotoTag=X_u  TagVisibility=global
  From3 : From  Commented=on  GotoTag=DCM_b2e  TagVisibility=global
  Gain : Gain  Commented=on
  Math Function1 : Math  Commented=on  Operator=transpose  SaturateOnIntegerOverflow=on
  N3 : Scope
  Selector1 : Selector  InputPortWidth=3  IndexOptions=Index vector (dialog)  Indices=[1 3]  OutputSizes=1
  Selector2 : Selector  Commented=on  InputPortWidth=3  IndexOptions=Index vector (dialog)  Indices=2  OutputSizes=1
  Selector6 : Selector  Commented=on  InputPortWidth=2  IndexOptions=Index vector (dialog)  Indices=2  OutputSizes=1
  Zero-Order Hold : ZeroOrderHold  SampleTime=-1
  magnitude : Subsystem
  V_wind : Outport
  omega_wind : Outport  Port=2
  wires:
  Selector6/1 -> Gain/1
  Gain/1 -> Dryden Wind Turbulence Model (Continuous (+q +r))/1
  Bias/1 -> Dryden Wind Turbulence Model (Continuous (+q +r))/2, Discrete Wind Gust Model/1
  Math Function1/1 -> Dryden Wind Turbulence Model (Continuous (+q +r))/3
  From3/1 -> Math Function1/1
  Dryden Wind Turbulence Model (Continuous (+q +r))/2 -> Selector2/1
  magnitude/1(Out1) -> Bias/1
  From25/1 -> Selector6/1
  [Xdot_u] -> magnitude/1(In1)
  Discrete Wind Gust Model/1 -> Selector1/1
  Selector1/1 -> Zero-Order Hold/1
  Selector2/1 -> omega_wind/1
  Zero-Order Hold/1 -> N3/1, V_wind/1

== system Marine_LocoMotive_UAV_est_git/Preprocessing Unit/Alpha_bar ==
  note: x_rel true
  note: Key to specify "front" or "rear" configuration.
  note: find desired x_rel and z_rel for the UAV:
      | x_rel_des = sqrt(r_bar^2 - (zu_bar-zb)^2)
      |
      | Note that the sign of x_rel is still anbiguous at this stage
  note: 1- Calculate alpha_bar based on x_rel and z_rel
  note: Z bar calculation during switching side mode:
      | (the UAV elevation changes from the reference hold).
      | This signal is used for monitoring purpose (not used by the controller)
  zb : Inport
  r_bar : Inport  Port=2
  zq_bar : Inport  Port=3
  alpha : Inport  Port=4
  decelerate : Inport  Port=5
  switch side : Inport  Port=6
  "  " : Trigonometry
  Delay1 : Delay  DelayLength=1
  Logical Operator1 : Logic  AllPortsSameDT=off  OutDataTypeStr=boolean
  Math Function : Math  Operator=magnitude^2  SaturateOnIntegerOverflow=on
  Math Function2 : Math  Operator=magnitude^2  SaturateOnIntegerOverflow=on
  Mux1 : Mux  Inputs=2
  Mux2 : Mux  Inputs=2
  Product2 : Product
  Sqrt : Sqrt  Operator=signedSqrt  SaturateOnIntegerOverflow=on
  Sum : Sum  Inputs=|+-
  Sum1 : Sum  Inputs=|+-
  Sum2 : Sum  Inputs=|++
  Switch1 : Switch  Criteria=u2 > Threshold
  Switch2 : Switch  Criteria=u2 > Threshold
  Unary Minus : UnaryMinus
  "alpha_bar " : Trigonometry  Operator=atan2
  decelerate2 : InportShadow  Port=5
  has moved past the buoy1 : simulink/Logic and Bit Operations/Compare To Constant  relop=>  const=pi/2  OutDataTypeStr=boolean
  r_bar1 : InportShadow  Port=2
  smooth switch : Subsystem
  x_rel des : Scope
  x_rel_amb : Scope
  z_bar_ss : Scope
  z_rel : Scope
  z_rel1 : Scope
  zb1 : InportShadow
  zq_bar1 : InportShadow  Port=3
  alpha_bar : Outport
  x_rel_bar : Outport  Port=2
  z_bar : Outport  Port=3
  tag scope: alpha_bar_step=global, x_rel=global, x_rel_amb=global, x_rel_final=global
  wires:
  [x_rel] -> "alpha_bar "/2  "x_rel"
  Sum/1 -> z_rel/1, [z_rel], Math Function2/1  "z_rel"
  zb/1 -> Sum/2
  Math Function2/1 -> Sum1/2
  zq_bar/1 -> Sum/1
  r_bar/1 -> Math Function/1
  Math Function/1 -> Sum1/1
  Sum1/1 -> Sqrt/1
  [x_rel_amb] -> Switch1/3, smooth switch/1(u 1), Unary Minus/1  "x_rel_des"
  alpha/1 -> has moved past the buoy1/1
  [z_rel] -> "alpha_bar "/1
  decelerate/1 -> Logical Operator1/2
  has moved past the buoy1/1 -> Logical Operator1/1
  Logical Operator1/1 -> Delay1/1
  switch side/1 -> Switch2/2
  zq_bar1/1 -> Switch2/3
  Switch2/1 -> Mux2/2, z_bar/1
  zb1/1 -> Sum2/1
  Sum2/1 -> Mux2/1, Switch2/1
  [alpha_bar_step] -> "  "/1
  "  "/1 -> Product2/1
  r_bar1/1 -> Product2/2
  Product2/1 -> Sum2/2
  Sqrt/1 -> x_rel_amb/1, [x_rel_amb]  "x_rel_des"
  Delay1/1 -> [rear]
  "alpha_bar "/1 -> z_rel1/1, alpha_bar/1, [alpha_bar_step]
  smooth switch/1(y) -> Mux1/1, x_rel_bar/1, [x_rel]  "x_rel"
  Mux2/1 -> z_bar_ss/1
  decelerate2/1 -> Switch1/2, smooth switch/3(switch)
  Switch1/1 -> Mux1/2, [x_rel_final]
  Unary Minus/1 -> smooth switch/2(u 2), Switch1/1
  Mux1/1 -> x_rel des/1

== system Marine_LocoMotive_UAV_est_git/Preprocessing Unit/Buoy immersed volume estimation ==
  note: Expected Immersed Volume (m^3)
      | (based on exact damping coefficient)
  note: Mean Immersed Volume (m^3)
      | (based on estimated damping coefficient)
  Constant : Constant  Value=(m_b+m_u)/rho_w
  Constant1 : Constant  Value=(m_b+m_u)/rho_w
  Constant2 : Constant  Value=rho_w*g
  Constant3 : Constant  Value=rho_w*g
  Constant4 : Constant  Value=0
  Constant5 : Constant  Value=Vol_b
  Constant6 : Constant
  Constant7 : Constant
  D11 1 : Scope
  D11 3 : Scope
  D_1 : Selector  NumberOfDimensions=2  InputPortWidth=2  IndexOptions=Index vector (dialog),Index vector (dialog)  Indices=1,1  OutputSizes=1,1
  D_21 : Selector  NumberOfDimensions=2  InputPortWidth=2  IndexOptions=Index vector (dialog),Index vector (dialog)  Indices=2,1  OutputSizes=1,1
  Dead Zone : DeadZone  Commented=on  LowerValue=80*pi/180  UpperValue=100*pi/180  SaturateOnIntegerOverflow=on
  Divide : Product  Inputs=*/
  IC1 : InitialCondition  Value=Delta_h*l_b*h_b + l_b*h_b^2/2
  Mux2 : Mux  Inputs=2
  Product : Product  Inputs=*/
  Product1 : Product  Inputs=*/*
  Product2 : Product  Inputs=*/
  Product3 : Product  Inputs=*/*
  Saturation1 : Saturate  UpperLimit=inf  LowerLimit=0.1*pi/180
  Saturation2 : Saturate  UpperLimit=60*pi/180  LowerLimit=0.1*pi/180
  Sum1 : Sum  Inputs=|++
  Sum2 : Sum  Inputs=|+-
  Sum3 : Sum  Inputs=|++
  Sum4 : Sum  Inputs=|+-
  Trigonometric Function : Trigonometry  Operator=tan
  Trigonometric Function1 : Trigonometry  Operator=tan
  V_immersed ratio : Scope
  Vol_im_expected : Outport
  Vol_im_mean : Outport  Port=2
  wires:
  [V_r_bar] -> Product1/1
  Constant1/1 -> Sum3/1
  Sum2/1 -> D11 1/1, Product1/3
  Constant3/1 -> Product3/2
  Constant4/1 -> Sum4/1
  D_21/1 -> Sum2/1
  [D_123] -> D_1/1
  [D_123] -> D_21/1
  D_1/1 -> Product/1
  Product2/1 -> Sum4/2
  Saturation2/1 -> Trigonometric Function1/1
  Product3/1 -> Sum3/2
  Product1/1 -> Sum1/2
  Sum4/1 -> D11 3/1, Product3/3
  Constant/1 -> Sum1/1
  [V_r_bar] -> Product3/1
  Product/1 -> Sum2/2
  Saturation1/1 -> Trigonometric Function/1
  [theta_bar] -> Saturation1/1
  Constant2/1 -> Product1/2
  [theta_bar] -> Saturation2/1
  Sum3/1 -> IC1/1
  Constant7/1 -> Product/2
  [D11_bar] -> Product2/1
  Constant6/1 -> Product2/2
  Sum1/1 -> Mux2/1, Vol_im_expected/1
  IC1/1 -> Mux2/2, Vol_im_mean/1
  Divide/1 -> V_immersed ratio/1
  Constant5/1 -> Divide/2
  Mux2/1 -> Divide/1

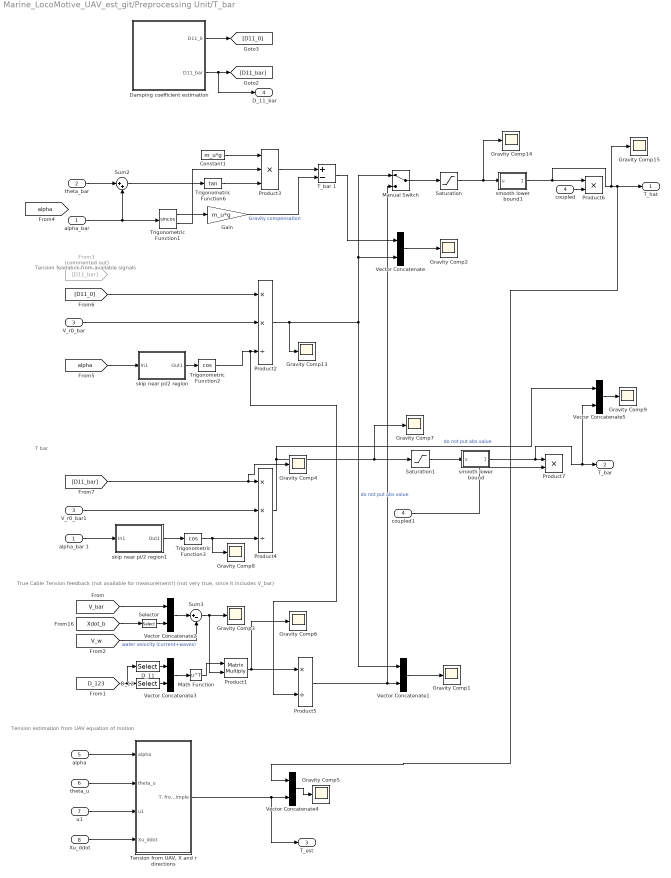
== system Marine_LocoMotive_UAV_est_git/Preprocessing Unit/T_bar  ==
  note: Tension feadabck from available signals
  note: True Cable Tension feedback (not available for measurement!) (not very true, since it includes V_bar)
  note: T bar
  note: Tension estimation from UAV equation of motion
  "alpha_bar " : Inport
  theta_bar : Inport  Port=2
  V_r0_bar : Inport  Port=3
  coupled : Inport  Port=4
  alpha : Inport  Port=5
  theta_u : Inport  Port=6
  u1 : Inport  Port=7
  Xu_ddot : Inport  Port=8
  Constant1 : Constant  Value=m_u*g
  D_11 : Selector  NumberOfDimensions=2  InputPortWidth=2  IndexOptions=Index vector (dialog),Index vector (dialog)  Indices=1,1  OutputSizes=1,1
  D_12 : Selector  NumberOfDimensions=2  InputPortWidth=2  IndexOptions=Index vector (dialog),Index vector (dialog)  Indices=1,2  OutputSizes=1,1
  Damping coefficient estimation : Subsystem
  From3 : From  Commented=on  GotoTag=D11_bar  TagVisibility=global
  Gain : Gain  Gain=m_u*g
  Gravity Comp{1..9,13..15} (12 alike) : Scope
  Manual Switch : ManualSwitch
  Math Function : Math  Operator=transpose  SaturateOnIntegerOverflow=on
  Product1 : Product  Multiplication=Matrix(*)
  Product2 : Product  Inputs=**/
  Product3 : Product  Inputs=***
  Product4 : Product  Inputs=**/
  Product5 : Product  Inputs=*/
  Product6 : Product
  Product7 : Product
  Saturation : Saturate  UpperLimit=inf  LowerLimit=epsilon_1
  Saturation1 : Saturate  UpperLimit=inf  LowerLimit=0
  Selector : Selector  InputPortWidth=2  IndexOptions=Index vector (dialog)  Indices=2  OutputSizes=1
  Sum2 : Sum  Inputs=|++
  Sum3 : Sum  Inputs=|+-
  T_bar 1 : Sum  Inputs=+-
  "Tension from UAV, X and r directions" : Subsystem
  Trigonometric Function1 : Trigonometry  Operator=sincos
  Trigonometric Function2 : Trigonometry  Operator=cos
  Trigonometric Function3 : Trigonometry  Operator=cos
  Trigonometric Function6 : Trigonometry  Operator=tan
  V_r0_bar1 : InportShadow  Port=3
  Vector Concatenate{,1..5} (6 alike) : Concatenate
  alpha_bar 1 : InportShadow
  coupled1 : InportShadow  Port=4
  skip near pi/2 region : Subsystem
  skip near pi/2 region1 : Subsystem
  smooth lower bound : Subsystem
  smooth lower bound1 : Subsystem
  T_hat : Outport
  T_bar : Outport  Port=2
  T_est : Outport  Port=3
  D_11_bar : Outport  Port=4
  wires:
  "alpha_bar "/1 -> Sum2/2, Trigonometric Function1/1
  Trigonometric Function1/1 -> Gain/1
  Gain/1 -> T_bar 1/2  "Gravity compensation"
  theta_bar/1 -> Sum2/1
  Sum2/1 -> Trigonometric Function6/1
  Vector Concatenate1/1 -> Gravity Comp1/1
  [D11_0] -> Product2/1
  Vector Concatenate/1 -> Gravity Comp2/1
  Constant1/1 -> Product3/1
  Trigonometric Function1/2 -> Product3/2
  Trigonometric Function6/1 -> Product3/3
  Product3/1 -> T_bar 1/1
  [D_123] -> D_11/1, D_12/1
  D_11/1 -> Vector Concatenate3/1
  [Xdot_b] -> Selector/1
  Sum3/1 -> Product1/2, Gravity Comp3/1
  Vector Concatenate2/1 -> Sum3/1
  [V_w] -> Sum3/2  "water velocity (current+waves)"
  Product1/1 -> Gravity Comp6/1, Product5/1
  Product5/1 -> Manual Switch/2, Vector Concatenate1/2
  Manual Switch/1 -> Saturation/1
  T_bar 1/1 -> Vector Concatenate/1
  Trigonometric Function2/1 -> Product5/2, Product2/3
  [V_bar] -> Vector Concatenate2/1
  Selector/1 -> Vector Concatenate2/2
  D_12/1 -> Vector Concatenate3/2
  Vector Concatenate3/1 -> Math Function/1
  Math Function/1 -> Product1/1
  alpha_bar 1/1 -> skip near pi/2 region1/1(In1)
  [D11_bar] -> Product4/1, Gravity Comp4/1
  Trigonometric Function3/1 -> Gravity Comp8/1, Product4/3
  Saturation/1 -> Gravity Comp14/1, smooth lower bound1/1(u)
  coupled/1 -> Product6/2
  Saturation1/1 -> smooth lower bound/1(u)
  skip near pi/2 region1/1(Out1) -> Trigonometric Function3/1
  theta_u/1 -> "Tension from UAV, X and r directions"/2(theta_u)
  alpha/1 -> "Tension from UAV, X and r directions"/1(alpha)
  Xu_ddot/1 -> "Tension from UAV, X and r directions"/4(Xu_ddot)
  u1/1 -> "Tension from UAV, X and r directions"/3(u1)
  Vector Concatenate4/1 -> Gravity Comp5/1
  Damping coefficient estimation/1(D11_0) -> [D11_0]
  Damping coefficient estimation/2(D11_bar) -> [D11_bar], D_11_bar/1
  coupled1/1 -> Product7/2
  smooth lower bound/1(sat(u)) -> Vector Concatenate5/2, T_bar/1, Product7/1
  V_r0_bar1/1 -> Product4/2
  Product4/1 -> Gravity Comp7/1, Saturation1/1, Vector Concatenate5/1  "do not put abs value"
  Vector Concatenate5/1 -> Gravity Comp9/1
  smooth lower bound1/1(sat(u)) -> Gravity Comp15/1, Vector Concatenate4/1, T_hat/1, Product6/1
  "Tension from UAV, X and r directions"/1("T, from x simple") -> T_est/1, Vector Concatenate4/2
  Product2/1 -> Manual Switch/1, Vector Concatenate/2, Vector Concatenate1/1, Gravity Comp13/1  "do not put abs value"
  V_r0_bar/1 -> Product2/2
  [alpha] -> skip near pi/2 region/1(In1)
  skip near pi/2 region/1(Out1) -> Trigonometric Function2/1

== system Marine_LocoMotive_UAV_est_git/Preprocessing Unit/Theta_bar  ==
  "alpha_bar " : Inport
  V_r0_bar : Inport  Port=2
  D11_bar : Inport  Port=3
  switch side1 : Inport  Port=4
  Add : Sum
  Constant : Constant  Value=alpha_bar
  D_11 : Selector  NumberOfDimensions=2  InputPortWidth=2  IndexOptions=Index vector (dialog),Index vector (dialog)  Indices=1,1  OutputSizes=1,1
  Gain : Gain  Gain=m_u*g
  Mux : Mux  Inputs=2
  Product1 : Product
  Product2 : Product  Inputs=**
  Product3 : Product
  Scope : Scope
  Switch : Switch  Criteria=u2 > Threshold
  Trigonometric Function3 : Trigonometry  Operator=sincos
  "theta_bar " : Trigonometry  Operator=atan2
  theta_bar : Outport
  wires:
  "theta_bar "/1 -> theta_bar/1
  "alpha_bar "/1 -> Switch/3
  Product1/1 -> "theta_bar "/1  "dy"
  Add/1 -> "theta_bar "/2  "dx"
  Product2/1 -> Add/1
  Trigonometric Function3/1 -> Product2/1
  Trigonometric Function3/2 -> Product1/2, Gain/1
  Gain/1 -> Add/2
  [D_123] -> D_11/1
  V_r0_bar/1 -> Product3/2
  Product3/1 -> Product2/2, Product1/1
  D11_bar/1 -> Mux/2, Product3/1
  Mux/1 -> Scope/1
  D_11/1 -> Mux/1
  switch side1/1 -> Switch/2
  Switch/1 -> Trigonometric Function3/1
  Constant/1 -> Switch/1
